simulink model "chap4_1sim"  (Simulink 6.3)
settings: Solver=ode3  StartTime=0.0  StopTime=20  FixedStep=0.001  RelTol=1e-3
settings Model: LastModifiedBy=Administrator

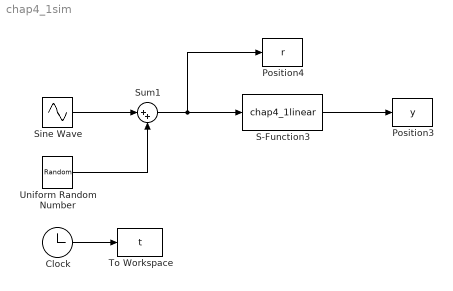
== system chap4_1sim ==
  Clock : Clock
      settings: Decimation=10
  Position3 : ToWorkspace  VariableName=y  SampleTime=-1  SaveFormat=Array
  Position4 : ToWorkspace  VariableName=r  SampleTime=-1  SaveFormat=Array
  S-Function3 : S-Function  FunctionName=chap4_1linear
  Sine Wave : Sin  SampleTime=0
  Sum1 : Sum  Inputs=|++
  To Workspace : ToWorkspace  VariableName=t  SampleTime=-1  SaveFormat=Array
  Uniform Random Number : UniformRandomNumber  Minimum=-0.05  Maximum=0.05  SampleTime=0
  wires:
  Sine Wave/1 -> Sum1/1
  Clock/1 -> To Workspace/1
  Uniform Random Number/1 -> Sum1/2
  Sum1/1 -> S-Function3/1, Position4/1
  S-Function3/1 -> Position3/1
